simulink model "Copy_of_AB_Final_of_MPC_Bandwidth_Result"  (R2022b)
settings: Solver=FixedStepDiscrete  StartTime=0.0  StopTime=Inf  FixedStep=100e-6  RelTol=1e-3  EnableMultiTasking=on
undefined symbols (not defined in the file): C28x, CPU1, CPU2, CurrentBypassValue, DiscIntNeverNeededParam, Down, GPTRIP1SEL, TZ1, Up
libraries: c2802xlib x31, simulink x22, dspstat3 x17, dspsigops x9, c2837xDlib x6, c280xlib x5, PID_Lib x2, c2000lib x1, spsAlphaBetaZerotoabcLib x1, spsAlphaBetaZerotodq0Lib x1
(part 4 of 8)

== system Copy_of_AB_Final_of_MPC_Bandwidth_Result/Subsystem1/AlphaBetaDutiesCalculation/DutiesCalculation ==
  MPCC_f32AlphaVoltageReference : Inport
  MPCC_f32BetaVoltageReference : Inport  Port=2
  MPCC_f32DCLinkVoltage : Inport  Port=3
  Duty_Sector1 : Subsystem
  Duty_Sector2 : Subsystem
  Duty_Sector3 : Subsystem
  Duty_Sector4 : Subsystem
  Duty_Sector5 : Subsystem
  Duty_Sector6 : Subsystem
  Gain : Gain  Gain=2/3
  Gain{1,4,17,22} (4 alike) : Gain  Gain=1/3
  Gain10 : Gain  Gain=-2/3
  Gain{2,11..12,19} (4 alike) : Gain  Gain=0
  Gain13 : Gain  Gain=-1/sqrt(3)
  Gain14 : Gain  Gain=-2/3
  Gain{5,8,15..16} (4 alike) : Gain  Gain=-1/3
  Gain18 : Gain  Gain=-1/sqrt(3)
  Gain21 : Gain  Gain=-1/sqrt(3)
  Gain23 : Gain  Gain=2/3
  Gain{3,6..7,9} (4 alike) : Gain  Gain=1/sqrt(3)
  MPCC_f32Duty_Sector1 : Outport
  MPCC_f32Duty_Sector2 : Outport  Port=2
  MPCC_f32Duty_Sector3 : Outport  Port=3
  MPCC_f32Duty_Sector4 : Outport  Port=4
  MPCC_f32Duty_Sector5 : Outport  Port=5
  MPCC_f32Duty_Sector6 : Outport  Port=6
  wires:
  Duty_Sector1/1(MPCC_f32Duty_Sector1) -> MPCC_f32Duty_Sector1/1
  MPCC_f32DCLinkVoltage/1 -> [MPCC_f32DCLinkVoltage]
  Gain/1 -> Duty_Sector1/3(MPCC_f32AlphaConvVoltage1)
  [MPCC_f32DCLinkVoltage] -> Gain2/1, Gain3/1, Gain1/1, Gain/1
  Gain1/1 -> Duty_Sector1/4(MPCC_f32AlphaConvVoltage2)
  Gain2/1 -> Duty_Sector1/5(MPCC_f32BetaConvVoltage1)
  Gain3/1 -> Duty_Sector1/6(MPCC_f32BetaConvVoltage2)
  Duty_Sector2/1(MPCC_f32Duty_Sector2) -> MPCC_f32Duty_Sector2/1
  Gain7/1 -> Duty_Sector2/6(MPCC_f32BetaConvVoltage3)
  Gain4/1 -> Duty_Sector2/3(MPCC_f32AlphaConvVoltage2)
  Gain5/1 -> Duty_Sector2/4(MPCC_f32AlphaConvVoltage3)
  [MPCC_f32DCLinkVoltage] -> Gain6/1, Gain7/1, Gain5/1, Gain4/1
  [MPCC_f32DCLinkVoltage] -> Gain11/1, Gain9/1, Gain10/1, Gain8/1
  Duty_Sector3/1(MPCC_f32Duty_Sector3) -> MPCC_f32Duty_Sector3/1
  Duty_Sector4/1(MPCC_f32Duty_Sector4) -> MPCC_f32Duty_Sector4/1
  Gain13/1 -> Duty_Sector4/6(MPCC_f32BetaConvVoltage5)
  [MPCC_f32DCLinkVoltage] -> Gain12/1, Gain13/1, Gain15/1, Gain14/1
  Duty_Sector5/1(MPCC_f32Duty_Sector5) -> MPCC_f32Duty_Sector5/1
  [MPCC_f32DCLinkVoltage] -> Gain18/1, Gain17/1, Gain16/1
  Duty_Sector6/1(MPCC_f32Duty_Sector6) -> MPCC_f32Duty_Sector6/1
  Gain21/1 -> Duty_Sector6/5(MPCC_f32BetaConvVoltage6)
  [MPCC_f32DCLinkVoltage] -> Gain19/1, Gain21/1, Gain23/1, Gain22/1
  MPCC_f32AlphaVoltageReference/1 -> [MPCC_f32AlphaVoltageReference]
  MPCC_f32BetaVoltageReference/1 -> [MPCC_f32BetaVoltageReference]
  [MPCC_f32AlphaVoltageReference] -> Duty_Sector1/1(MPCC_f32AlphaVoltageReference)
  [MPCC_f32BetaVoltageReference] -> Duty_Sector1/2(MPCC_f32BetaVoltageReference)
  [MPCC_f32AlphaVoltageReference] -> Duty_Sector2/1(MPCC_f32AlphaVoltageReference)
  [MPCC_f32BetaVoltageReference] -> Duty_Sector2/2(MPCC_f32BetaVoltageReference)
  [MPCC_f32AlphaVoltageReference] -> Duty_Sector3/1(MPCC_f32AlphaVoltageReference)
  [MPCC_f32BetaVoltageReference] -> Duty_Sector3/2(MPCC_f32BetaVoltageReference)
  [MPCC_f32AlphaVoltageReference] -> Duty_Sector4/1(MPCC_f32AlphaVoltageReference)
  [MPCC_f32BetaVoltageReference] -> Duty_Sector4/2(MPCC_f32BetaVoltageReference)
  [MPCC_f32AlphaVoltageReference] -> Duty_Sector5/1(MPCC_f32AlphaVoltageReference)
  [MPCC_f32BetaVoltageReference] -> Duty_Sector5/2(MPCC_f32BetaVoltageReference)
  [MPCC_f32AlphaVoltageReference] -> Duty_Sector6/1(MPCC_f32AlphaVoltageReference)
  [MPCC_f32BetaVoltageReference] -> Duty_Sector6/2(MPCC_f32BetaVoltageReference)
  Gain6/1 -> Duty_Sector2/5(MPCC_f32BetaConvVoltage2)
  Gain8/1 -> Duty_Sector3/3(MPCC_f32AlphaConvVoltage3)
  Gain9/1 -> Duty_Sector3/5(MPCC_f32BetaConvVoltage3)
  Gain10/1 -> Duty_Sector3/4(MPCC_f32AlphaConvVoltage4)
  Gain11/1 -> Duty_Sector3/6(MPCC_f32BetaConvVoltage4)
  Gain14/1 -> Duty_Sector4/3(MPCC_f32AlphaConvVoltage4)
  Gain12/1 -> Duty_Sector4/5(MPCC_f32BetaConvVoltage4)
  Gain15/1 -> Duty_Sector4/4(MPCC_f32AlphaConvVoltage5)
  Gain18/1 -> Duty_Sector5/5(MPCC_f32BetaConvVoltage5), Duty_Sector5/6(MPCC_f32BetaConvVoltage6)
  Gain16/1 -> Duty_Sector5/3(MPCC_f32AlphaConvVoltage5)
  Gain17/1 -> Duty_Sector5/4(MPCC_f32AlphaConvVoltage6)
  Gain22/1 -> Duty_Sector6/3(MPCC_f32AlphaConvVoltage6)
  Gain23/1 -> Duty_Sector6/4(MPCC_f32AlphaConvVoltage1)
  Gain19/1 -> Duty_Sector6/6(MPCC_f32BetaConvVoltage1)

== system Copy_of_AB_Final_of_MPC_Bandwidth_Result/Subsystem1/GridCurrentFirstPrediction/PredictedIdGridCurrentCalculation ==
  MPCC_f32Predictionterm_A : Inport
  MPCC_f32Predictionterm_B : Inport  Port=2
  MPCC_f32Predictionterm_C : Inport  Port=3
  MPCC_f32DGridCurrent : Inport  Port=4
  MPCC_f32QGridCurrent : Inport  Port=5
  MPCC_f32DGridVoltage : Inport  Port=6
  MPCC_f32DConvVoltage : Inport  Port=7
  Add : Sum  Inputs=+++-
  Gain : Gain  Gain=0
  Product{,1..2,4} (4 alike) : Product
  MPCC_f32DGridCurrent_K_1 : Outport
  wires:
  Product/1 -> Add/1
  [MPCC_f32QGridCurrent] -> Product1/2
  [MPCC_f32Predictionterm_A] -> Product/1
  Product1/1 -> Gain/1
  [MPCC_f32DGridVoltage] -> Product2/2
  [MPCC_f32DGridCurrent] -> Product/2
  [MPCC_f32Predictionterm_C] -> Product1/1
  [MPCC_f32Predictionterm_B] -> Product2/1
  MPCC_f32Predictionterm_A/1 -> [MPCC_f32Predictionterm_A]
  MPCC_f32Predictionterm_B/1 -> [MPCC_f32Predictionterm_B]
  MPCC_f32Predictionterm_C/1 -> [MPCC_f32Predictionterm_C]
  MPCC_f32DGridCurrent/1 -> [MPCC_f32DGridCurrent]
  MPCC_f32QGridCurrent/1 -> [MPCC_f32QGridCurrent]
  MPCC_f32DGridVoltage/1 -> [MPCC_f32DGridVoltage]
  MPCC_f32DConvVoltage/1 -> [MPCC_f32DConvVoltage]
  Add/1 -> MPCC_f32DGridCurrent_K_1/1
  [MPCC_f32Predictionterm_B] -> Product4/1
  [MPCC_f32DConvVoltage] -> Product4/2
  Product2/1 -> Add/3
  Product4/1 -> Add/4
  Gain/1 -> Add/2

== system Copy_of_AB_Final_of_MPC_Bandwidth_Result/Subsystem1/GridCurrentFirstPrediction/PredictedIqGridCurrentCalculation ==
  MPCC_f32Predictionterm_A : Inport
  MPCC_f32Predictionterm_B : Inport  Port=2
  MPCC_f32Predictionterm_C : Inport  Port=3
  MPCC_f32DGridCurrent : Inport  Port=4
  MPCC_f32QGridCurrent : Inport  Port=5
  MPCC_f32QGridVoltage : Inport  Port=6
  MPCC_f32QConvVoltage : Inport  Port=7
  Add : Sum  Inputs=+-+-
  Gain : Gain  Gain=0
  Product : Product  OutDataTypeStr=Inherit: Inherit via back propagation
  Product1 : Product
  Product2 : Product
  Product4 : Product
  MPCC_f32QVoltageReference : Outport
  wires:
  Product/1 -> Add/1
  [MPCC_f32DGridCurrent] -> Product1/2
  [MPCC_f32Predictionterm_A] -> Product/1
  Product1/1 -> Gain/1
  [MPCC_f32QGridVoltage] -> Product2/2
  [MPCC_f32QGridCurrent] -> Product/2
  [MPCC_f32Predictionterm_C] -> Product1/1
  [MPCC_f32Predictionterm_B] -> Product2/1
  MPCC_f32Predictionterm_A/1 -> [MPCC_f32Predictionterm_A]
  MPCC_f32Predictionterm_B/1 -> [MPCC_f32Predictionterm_B]
  MPCC_f32Predictionterm_C/1 -> [MPCC_f32Predictionterm_C]
  MPCC_f32DGridCurrent/1 -> [MPCC_f32DGridCurrent]
  MPCC_f32QGridCurrent/1 -> [MPCC_f32QGridCurrent]
  MPCC_f32QGridVoltage/1 -> [MPCC_f32QGridVoltage]
  MPCC_f32QConvVoltage/1 -> [MPCC_f32QConvVoltage]
  Add/1 -> MPCC_f32QVoltageReference/1
  [MPCC_f32Predictionterm_B] -> Product4/1
  [MPCC_f32QConvVoltage] -> Product4/2
  Product2/1 -> Add/3
  Product4/1 -> Add/4
  Gain/1 -> Add/2

== system Copy_of_AB_Final_of_MPC_Bandwidth_Result/Subsystem1/GridCurrentSecondPrediction/CostFunctionofSectors ==
  MPCC_f32CostFunction_Voltage1 : Inport
  MPCC_f32CostFunction_Voltage2 : Inport  Port=2
  MPCC_f32CostFunction_Voltage3 : Inport  Port=3
  MPCC_f32CostFunction_Voltage4 : Inport  Port=4
  MPCC_f32CostFunction_Voltage5 : Inport  Port=5
  MPCC_f32CostFunction_Voltage6 : Inport  Port=6
  MPCC_f32Duty_Sector1 : Inport  Port=7
  MPCC_f32Duty_Sector2 : Inport  Port=8
  MPCC_f32Duty_Sector3 : Inport  Port=9
  MPCC_f32Duty_Sector4 : Inport  Port=10
  MPCC_f32Duty_Sector5 : Inport  Port=11
  MPCC_f32Duty_Sector6 : Inport  Port=12
  Duty_Sector1 : Subsystem
  Duty_Sector2 : Subsystem
  Duty_Sector3 : Subsystem
  Duty_Sector4 : Subsystem
  Duty_Sector5 : Subsystem
  Duty_Sector6 : Subsystem
  MPCC_f32CostFunction_Sector1 : Outport
  MPCC_f32CostFunction_Sector2 : Outport  Port=2
  MPCC_f32CostFunction_Sector3 : Outport  Port=3
  MPCC_f32CostFunction_Sector4 : Outport  Port=4
  MPCC_f32CostFunction_Sector5 : Outport  Port=5
  MPCC_f32CostFunction_Sector6 : Outport  Port=6
  wires:
  Duty_Sector1/1(MPCC_f32CostFunction_Sector1) -> MPCC_f32CostFunction_Sector1/1
  [MPCC_f32CostFunction_Voltage1] -> Duty_Sector1/1(MPCC_f32CostFunction_Voltage1)
  [MPCC_f32CostFunction_Voltage2] -> Duty_Sector1/2(MPCC_f32CostFunction_Voltage2)
  [MPCC_f32Duty_Sector1] -> Duty_Sector1/3(MPCC_f32Duty_Sector1)
  MPCC_f32Duty_Sector1/1 -> [MPCC_f32Duty_Sector1]
  MPCC_f32CostFunction_Voltage1/1 -> [MPCC_f32CostFunction_Voltage1]
  MPCC_f32CostFunction_Voltage2/1 -> [MPCC_f32CostFunction_Voltage2]
  MPCC_f32CostFunction_Voltage3/1 -> [MPCC_f32CostFunction_Voltage3]
  MPCC_f32CostFunction_Voltage4/1 -> [MPCC_f32CostFunction_Voltage4]
  MPCC_f32CostFunction_Voltage5/1 -> [MPCC_f32CostFunction_Voltage5]
  MPCC_f32CostFunction_Voltage6/1 -> [MPCC_f32CostFunction_Voltage6]
  MPCC_f32Duty_Sector2/1 -> [MPCC_f32Duty_Sector2]
  MPCC_f32Duty_Sector3/1 -> [MPCC_f32Duty_Sector3]
  MPCC_f32Duty_Sector4/1 -> [MPCC_f32Duty_Sector4]
  MPCC_f32Duty_Sector5/1 -> [MPCC_f32Duty_Sector5]
  MPCC_f32Duty_Sector6/1 -> [MPCC_f32Duty_Sector6]
  Duty_Sector2/1(MPCC_f32CostFunction_Sector2) -> MPCC_f32CostFunction_Sector2/1
  [MPCC_f32Duty_Sector2] -> Duty_Sector2/3(MPCC_f32Duty_Sector2)
  [MPCC_f32CostFunction_Voltage3] -> Duty_Sector2/2(MPCC_f32CostFunction_Voltage3)
  [MPCC_f32CostFunction_Voltage2] -> Duty_Sector2/1(MPCC_f32CostFunction_Voltage2)
  [MPCC_f32CostFunction_Voltage4] -> Duty_Sector3/2(MPCC_f32CostFunction_Voltage4)
  [MPCC_f32CostFunction_Voltage3] -> Duty_Sector3/1(MPCC_f32CostFunction_Voltage3)
  Duty_Sector3/1(MPCC_f32CostFunction_Sector3) -> MPCC_f32CostFunction_Sector3/1
  [MPCC_f32Duty_Sector3] -> Duty_Sector3/3(MPCC_f32Duty_Sector3)
  [MPCC_f32CostFunction_Voltage4] -> Duty_Sector4/1(MPCC_f32CostFunction_Voltage4)
  Duty_Sector4/1(MPCC_f32CostFunction_Sector4) -> MPCC_f32CostFunction_Sector4/1
  [MPCC_f32Duty_Sector4] -> Duty_Sector4/3(MPCC_f32Duty_Sector4)
  [MPCC_f32CostFunction_Voltage5] -> Duty_Sector4/2(MPCC_f32CostFunction_Voltage5)
  [MPCC_f32CostFunction_Voltage5] -> Duty_Sector5/1(MPCC_f32CostFunction_Voltage5)
  [MPCC_f32Duty_Sector5] -> Duty_Sector5/3(MPCC_f32Duty_Sector5)
  Duty_Sector5/1(MPCC_f32CostFunction_Sector5) -> MPCC_f32CostFunction_Sector5/1
  [MPCC_f32CostFunction_Voltage6] -> Duty_Sector5/2(MPCC_f32CostFunction_Voltage6)
  [MPCC_f32CostFunction_Voltage1] -> Duty_Sector6/2(MPCC_f32CostFunction_Voltage1)
  [MPCC_f32Duty_Sector6] -> Duty_Sector6/3(MPCC_f32Duty_Sector6)
  Duty_Sector6/1(MPCC_f32CostFunction_Sector6) -> MPCC_f32CostFunction_Sector6/1
  [MPCC_f32CostFunction_Voltage6] -> Duty_Sector6/1(MPCC_f32CostFunction_Voltage6)

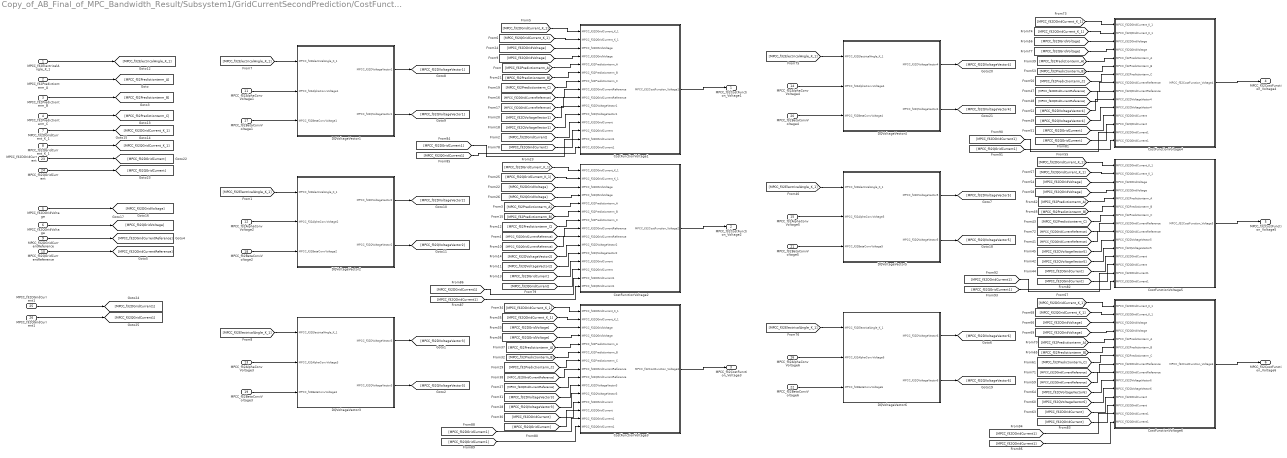
== system Copy_of_AB_Final_of_MPC_Bandwidth_Result/Subsystem1/GridCurrentSecondPrediction/CostFunctionofVoltageVectors ==
  MPCC_f32ElectricalAngle_K_1 : Inport
  MPCC_f32Predictionterm_A : Inport  Port=2
  MPCC_f32Predictionterm_B : Inport  Port=3
  MPCC_f32Predictionterm_C : Inport  Port=4
  MPCC_f32DGridVoltage : Inport  Port=5
  MPCC_f32QGridVoltage : Inport  Port=6
  MPCC_f32DGridCurrent_K_1 : Inport  Port=7
  MPCC_f32QGridCurrent_K_1 : Inport  Port=8
  MPCC_f32DGridCurrentReference : Inport  Port=9
  MPCC_f32QGridCurrentReference : Inport  Port=10
  MPCC_f32AlphaConvVoltage1 : Inport  Port=11
  MPCC_f32AlphaConvVoltage2 : Inport  Port=12
  MPCC_f32AlphaConvVoltage3 : Inport  Port=13
  MPCC_f32AlphaConvVoltage4 : Inport  Port=14
  MPCC_f32AlphaConvVoltage5 : Inport  Port=15
  MPCC_f32AlphaConvVoltage6 : Inport  Port=16
  MPCC_f32BetaConvVoltage1 : Inport  Port=17
  MPCC_f32BetaConvVoltage2 : Inport  Port=18
  MPCC_f32BetaConvVoltage3 : Inport  Port=19
  MPCC_f32BetaConvVoltage4 : Inport  Port=20
  MPCC_f32BetaConvVoltage5 : Inport  Port=21
  MPCC_f32BetaConvVoltage6 : Inport  Port=22
  MPCC_f32DGridCurrent : Inport  Port=23
  MPCC_f32QGridCurrent : Inport  Port=24
  MPCC_f32DGridCurrent1 : Inport  Port=25
  MPCC_f32QGridCurrent1 : Inport  Port=26
  CostFunctionVoltage1 : Subsystem
  CostFunctionVoltage2 : Subsystem
  CostFunctionVoltage3 : Subsystem
  CostFunctionVoltage4 : Subsystem
  CostFunctionVoltage5 : Subsystem
  CostFunctionVoltage6 : Subsystem
  DQVoltageVector1 : Subsystem
  DQVoltageVector2 : Subsystem
  DQVoltageVector3 : Subsystem
  DQVoltageVector4 : Subsystem
  DQVoltageVector5 : Subsystem
  DQVoltageVector6 : Subsystem
  MPCC_f32CostFunction_Voltage1 : Outport
  MPCC_f32CostFunction_Voltage2 : Outport  Port=2
  MPCC_f32CostFunction_Voltage3 : Outport  Port=3
  MPCC_f32CostFunction_Voltage4 : Outport  Port=4
  MPCC_f32CostFunction_Voltage5 : Outport  Port=5
  MPCC_f32CostFunction_Voltage6 : Outport  Port=6
  wires:
  DQVoltageVector1/1(MPCC_f32DVoltageVector1) -> [MPCC_f32DVoltageVector1]
  DQVoltageVector1/2(MPCC_f32QVoltageVector1) -> [MPCC_f32QVoltageVector1]
  DQVoltageVector2/1(MPCC_f32DVoltageVector2) -> [MPCC_f32DVoltageVector2]
  DQVoltageVector2/2(MPCC_f32QVoltageVector2) -> [MPCC_f32QVoltageVector2]
  [MPCC_f32ElectricalAngle_K_1] -> DQVoltageVector1/1(MPCC_f32ElectricalAngle_K_1)
  [MPCC_f32ElectricalAngle_K_1] -> DQVoltageVector2/1(MPCC_f32ElectricalAngle_K_1)
  MPCC_f32AlphaConvVoltage1/1 -> DQVoltageVector1/2(MPCC_f32AlphaConvVoltage1)
  MPCC_f32BetaConvVoltage1/1 -> DQVoltageVector1/3(MPCC_f32BetaConvVoltage1)
  MPCC_f32AlphaConvVoltage2/1 -> DQVoltageVector2/2(MPCC_f32AlphaConvVoltage2)
  MPCC_f32BetaConvVoltage2/1 -> DQVoltageVector2/3(MPCC_f32BetaConvVoltage2)
  MPCC_f32ElectricalAngle_K_1/1 -> [MPCC_f32ElectricalAngle_K_1]
  MPCC_f32DGridVoltage/1 -> [MPCC_f32DGridVoltage]
  MPCC_f32QGridCurrent_K_1/1 -> [MPCC_f32QGridCurrent_K_1]
  MPCC_f32DGridCurrent_K_1/1 -> [MPCC_f32DGridCurrent_K_1]
  MPCC_f32QGridVoltage/1 -> [MPCC_f32QGridVoltage]
  MPCC_f32Predictionterm_B/1 -> [MPCC_f32Predictionterm_B]
  MPCC_f32Predictionterm_C/1 -> [MPCC_f32Predictionterm_C]
  MPCC_f32Predictionterm_A/1 -> [MPCC_f32Predictionterm_A]
  MPCC_f32DGridCurrentReference/1 -> [MPCC_f32DGridCurrentReference]
  MPCC_f32QGridCurrentReference/1 -> [MPCC_f32QGridCurrentReference]
  CostFunctionVoltage1/1(MPCC_f32CostFunction_Voltage1) -> MPCC_f32CostFunction_Voltage1/1
  CostFunctionVoltage2/1(MPCC_f32CostFunction_Voltage2) -> MPCC_f32CostFunction_Voltage2/1
  [MPCC_f32DGridCurrent_K_1] -> CostFunctionVoltage1/1(MPCC_f32DGridCurrent_K_1)
  [MPCC_f32QGridCurrent_K_1] -> CostFunctionVoltage1/2(MPCC_f32QGridCurrent_K_1)
  [MPCC_f32DGridVoltage] -> CostFunctionVoltage1/3(MPCC_f32DGridVoltage)
  [MPCC_f32QGridVoltage] -> CostFunctionVoltage1/4(MPCC_f32QGridVoltage)
  [MPCC_f32Predictionterm_A] -> CostFunctionVoltage1/5(MPCC_f32Predictionterm_A)
  [MPCC_f32Predictionterm_B] -> CostFunctionVoltage1/6(MPCC_f32Predictionterm_B)
  [MPCC_f32Predictionterm_C] -> CostFunctionVoltage1/7(MPCC_f32Predictionterm_C)
  [MPCC_f32DGridCurrentReference] -> CostFunctionVoltage1/8(MPCC_f32DGridCurrentReference)
  [MPCC_f32QGridCurrentReference] -> CostFunctionVoltage1/9(MPCC_f32QGridCurrentReference)
  [MPCC_f32DVoltageVector1] -> CostFunctionVoltage1/10(MPCC_f32DVoltageVector1)
  [MPCC_f32QVoltageVector1] -> CostFunctionVoltage1/11(MPCC_f32QVoltageVector1)
  [MPCC_f32Predictionterm_C] -> CostFunctionVoltage2/7(MPCC_f32Predictionterm_C)
  [MPCC_f32DGridCurrentReference] -> CostFunctionVoltage2/8(MPCC_f32DGridCurrentReference)
  [MPCC_f32QGridCurrentReference] -> CostFunctionVoltage2/9(MPCC_f32QGridCurrentReference)
  [MPCC_f32DVoltageVector2] -> CostFunctionVoltage2/10(MPCC_f32DVoltageVector2)
  [MPCC_f32QVoltageVector2] -> CostFunctionVoltage2/11(MPCC_f32QVoltageVector2)
  [MPCC_f32QGridCurrent_K_1] -> CostFunctionVoltage2/2(MPCC_f32QGridCurrent_K_1)
  [MPCC_f32DGridVoltage] -> CostFunctionVoltage2/3(MPCC_f32DGridVoltage)
  [MPCC_f32QGridVoltage] -> CostFunctionVoltage2/4(MPCC_f32QGridVoltage)
  [MPCC_f32Predictionterm_A] -> CostFunctionVoltage2/5(MPCC_f32Predictionterm_A)
  [MPCC_f32Predictionterm_B] -> CostFunctionVoltage2/6(MPCC_f32Predictionterm_B)
  [MPCC_f32DGridCurrent_K_1] -> CostFunctionVoltage2/1(MPCC_f32DGridCurrent_K_1)
  MPCC_f32BetaConvVoltage3/1 -> DQVoltageVector3/3(MPCC_f32BetaConvVoltage3)
  MPCC_f32AlphaConvVoltage3/1 -> DQVoltageVector3/2(MPCC_f32AlphaConvVoltage3)
  [MPCC_f32ElectricalAngle_K_1] -> DQVoltageVector3/1(MPCC_f32ElectricalAngle_K_1)
  DQVoltageVector3/1(MPCC_f32DVoltageVector3) -> [MPCC_f32DVoltageVector3]
  DQVoltageVector3/2(MPCC_f32QVoltageVector3) -> [MPCC_f32QVoltageVector3]
  CostFunctionVoltage3/1(MPCC_f32CostFunction_Voltage3) -> MPCC_f32CostFunction_Voltage3/1
  [MPCC_f32Predictionterm_A] -> CostFunctionVoltage3/5(MPCC_f32Predictionterm_A)
  [MPCC_f32QGridVoltage] -> CostFunctionVoltage3/4(MPCC_f32QGridVoltage)
  [MPCC_f32Predictionterm_B] -> CostFunctionVoltage3/6(MPCC_f32Predictionterm_B)
  [MPCC_f32QGridCurrent_K_1] -> CostFunctionVoltage3/2(MPCC_f32QGridCurrent_K_1)
  [MPCC_f32QVoltageVector3] -> CostFunctionVoltage3/11(MPCC_f32QVoltageVector3)
  [MPCC_f32DVoltageVector3] -> CostFunctionVoltage3/10(MPCC_f32DVoltageVector3)
  [MPCC_f32DGridVoltage] -> CostFunctionVoltage3/3(MPCC_f32DGridVoltage)
  [MPCC_f32Predictionterm_C] -> CostFunctionVoltage3/7(MPCC_f32Predictionterm_C)
  [MPCC_f32QGridCurrentReference] -> CostFunctionVoltage3/9(MPCC_f32QGridCurrentReference)
  [MPCC_f32DGridCurrent_K_1] -> CostFunctionVoltage3/1(MPCC_f32DGridCurrent_K_1)
  [MPCC_f32DGridCurrentReference] -> CostFunctionVoltage3/8(MPCC_f32DGridCurrentReference)
  [MPCC_f32DGridVoltage] -> CostFunctionVoltage4/3(MPCC_f32DGridVoltage)
  [MPCC_f32Predictionterm_C] -> CostFunctionVoltage4/7(MPCC_f32Predictionterm_C)
  [MPCC_f32Predictionterm_B] -> CostFunctionVoltage4/6(MPCC_f32Predictionterm_B)
  [MPCC_f32QGridCurrent_K_1] -> CostFunctionVoltage4/2(MPCC_f32QGridCurrent_K_1)
  [MPCC_f32DGridCurrent_K_1] -> CostFunctionVoltage4/1(MPCC_f32DGridCurrent_K_1)
  [MPCC_f32Predictionterm_A] -> CostFunctionVoltage4/5(MPCC_f32Predictionterm_A)
  [MPCC_f32QGridVoltage] -> CostFunctionVoltage5/4(MPCC_f32QGridVoltage)
  [MPCC_f32Predictionterm_B] -> CostFunctionVoltage5/6(MPCC_f32Predictionterm_B)
  [MPCC_f32QGridCurrent_K_1] -> CostFunctionVoltage5/2(MPCC_f32QGridCurrent_K_1)
  [MPCC_f32DVoltageVector5] -> CostFunctionVoltage5/10(MPCC_f32DVoltageVector5)
  [MPCC_f32Predictionterm_C] -> CostFunctionVoltage5/7(MPCC_f32Predictionterm_C)
  [MPCC_f32DGridCurrentReference] -> CostFunctionVoltage5/8(MPCC_f32DGridCurrentReference)
  [MPCC_f32QGridCurrentReference] -> CostFunctionVoltage5/9(MPCC_f32QGridCurrentReference)
  [MPCC_f32DGridCurrent_K_1] -> CostFunctionVoltage5/1(MPCC_f32DGridCurrent_K_1)
  [MPCC_f32DVoltageVector4] -> CostFunctionVoltage4/10(MPCC_f32DVoltageVector4)
  [MPCC_f32QGridCurrentReference] -> CostFunctionVoltage6/9(MPCC_f32QGridCurrentReference)
  [MPCC_f32QVoltageVector5] -> CostFunctionVoltage5/11(MPCC_f32QVoltageVector5)
  [MPCC_f32DGridCurrentReference] -> CostFunctionVoltage6/8(MPCC_f32DGridCurrentReference)
  CostFunctionVoltage4/1(MPCC_f32CostFunction_Voltage4) -> MPCC_f32CostFunction_Voltage4/1
  [MPCC_f32DVoltageVector6] -> CostFunctionVoltage6/10(MPCC_f32DVoltageVector6)
  [MPCC_f32DGridVoltage] -> CostFunctionVoltage6/3(MPCC_f32DGridVoltage)
  [MPCC_f32Predictionterm_C] -> CostFunctionVoltage6/7(MPCC_f32Predictionterm_C)
  [MPCC_f32QGridVoltage] -> CostFunctionVoltage4/4(MPCC_f32QGridVoltage)
  [MPCC_f32QGridCurrent_K_1] -> CostFunctionVoltage6/2(MPCC_f32QGridCurrent_K_1)
  [MPCC_f32QVoltageVector6] -> CostFunctionVoltage6/11(MPCC_f32QVoltageVector6)
  [MPCC_f32Predictionterm_B] -> CostFunctionVoltage6/6(MPCC_f32Predictionterm_B)
  CostFunctionVoltage5/1(MPCC_f32CostFunction_Voltage5) -> MPCC_f32CostFunction_Voltage5/1
  [MPCC_f32QGridVoltage] -> CostFunctionVoltage6/4(MPCC_f32QGridVoltage)
  MPCC_f32AlphaConvVoltage6/1 -> DQVoltageVector6/2(MPCC_f32AlphaConvVoltage6)
  [MPCC_f32Predictionterm_A] -> CostFunctionVoltage5/5(MPCC_f32Predictionterm_A)
  DQVoltageVector6/1(MPCC_f32DVoltageVector6) -> [MPCC_f32DVoltageVector6]
  [MPCC_f32DGridVoltage] -> CostFunctionVoltage5/3(MPCC_f32DGridVoltage)
  MPCC_f32BetaConvVoltage6/1 -> DQVoltageVector6/3(MPCC_f32BetaConvVoltage6)
  DQVoltageVector6/2(MPCC_f32QVoltageVector6) -> [MPCC_f32QVoltageVector6]
  [MPCC_f32ElectricalAngle_K_1] -> DQVoltageVector4/1(MPCC_f32ElectricalAngle_K_1)
  DQVoltageVector5/2(MPCC_f32QVoltageVector5) -> [MPCC_f32QVoltageVector5]
  CostFunctionVoltage6/1(MPCC_f32CostFunction_Voltage6) -> MPCC_f32CostFunction_Voltage6/1
  MPCC_f32AlphaConvVoltage5/1 -> DQVoltageVector5/2(MPCC_f32AlphaConvVoltage5)
  DQVoltageVector4/1(MPCC_f32DVoltageVector4) -> [MPCC_f32DVoltageVector4]
  [MPCC_f32Predictionterm_A] -> CostFunctionVoltage6/5(MPCC_f32Predictionterm_A)
  DQVoltageVector4/2(MPCC_f32QVoltageVector4) -> [MPCC_f32QVoltageVector4]
  [MPCC_f32ElectricalAngle_K_1] -> DQVoltageVector5/1(MPCC_f32ElectricalAngle_K_1)
  MPCC_f32BetaConvVoltage4/1 -> DQVoltageVector4/3(MPCC_f32BetaConvVoltage4)
  [MPCC_f32QVoltageVector4] -> CostFunctionVoltage4/11(MPCC_f32QVoltageVector4)
  DQVoltageVector5/1(MPCC_f32DVoltageVector5) -> [MPCC_f32DVoltageVector5]
  [MPCC_f32QGridCurrentReference] -> CostFunctionVoltage4/9(MPCC_f32QGridCurrentReference)
  [MPCC_f32ElectricalAngle_K_1] -> DQVoltageVector6/1(MPCC_f32ElectricalAngle_K_1)
  [MPCC_f32DGridCurrent_K_1] -> CostFunctionVoltage6/1(MPCC_f32DGridCurrent_K_1)
  MPCC_f32AlphaConvVoltage4/1 -> DQVoltageVector4/2(MPCC_f32AlphaConvVoltage4)
  MPCC_f32BetaConvVoltage5/1 -> DQVoltageVector5/3(MPCC_f32BetaConvVoltage5)
  [MPCC_f32DGridCurrentReference] -> CostFunctionVoltage4/8(MPCC_f32DGridCurrentReference)
  [MPCC_f32DGridCurrent] -> CostFunctionVoltage1/12(MPCC_f32DGridCurrent)
  [MPCC_f32QGridCurrent] -> CostFunctionVoltage1/13(MPCC_f32QGridCurrent)
  MPCC_f32DGridCurrent/1 -> [MPCC_f32DGridCurrent]
  MPCC_f32QGridCurrent/1 -> [MPCC_f32QGridCurrent]
  [MPCC_f32DGridCurrent] -> CostFunctionVoltage2/12(MPCC_f32DGridCurrent)
  [MPCC_f32QGridCurrent] -> CostFunctionVoltage2/13(MPCC_f32QGridCurrent)
  [MPCC_f32DGridCurrent] -> CostFunctionVoltage3/12(MPCC_f32DGridCurrent)
  [MPCC_f32QGridCurrent] -> CostFunctionVoltage3/13(MPCC_f32QGridCurrent)
  [MPCC_f32DGridCurrent] -> CostFunctionVoltage4/12(MPCC_f32DGridCurrent)
  [MPCC_f32QGridCurrent] -> CostFunctionVoltage4/13(MPCC_f32QGridCurrent)
  [MPCC_f32DGridCurrent] -> CostFunctionVoltage5/12(MPCC_f32DGridCurrent)
  [MPCC_f32QGridCurrent] -> CostFunctionVoltage5/13(MPCC_f32QGridCurrent)
  [MPCC_f32DGridCurrent] -> CostFunctionVoltage6/12(MPCC_f32DGridCurrent)
  [MPCC_f32QGridCurrent] -> CostFunctionVoltage6/13(MPCC_f32QGridCurrent)
  MPCC_f32QGridCurrent1/1 -> [MPCC_f32QGridCurrent1]
  MPCC_f32DGridCurrent1/1 -> [MPCC_f32DGridCurrent1]
  [MPCC_f32DGridCurrent1] -> CostFunctionVoltage1/14(MPCC_f32DGridCurrent1)
  [MPCC_f32QGridCurrent1] -> CostFunctionVoltage1/15(MPCC_f32QGridCurrent1)
  [MPCC_f32DGridCurrent1] -> CostFunctionVoltage2/14(MPCC_f32DGridCurrent1)
  [MPCC_f32QGridCurrent1] -> CostFunctionVoltage2/15(MPCC_f32QGridCurrent1)
  [MPCC_f32DGridCurrent1] -> CostFunctionVoltage3/14(MPCC_f32DGridCurrent1)
  [MPCC_f32QGridCurrent1] -> CostFunctionVoltage3/15(MPCC_f32QGridCurrent1)
  [MPCC_f32DGridCurrent1] -> CostFunctionVoltage4/14(MPCC_f32DGridCurrent1)
  [MPCC_f32QGridCurrent1] -> CostFunctionVoltage4/15(MPCC_f32QGridCurrent1)
  [MPCC_f32DGridCurrent1] -> CostFunctionVoltage5/14(MPCC_f32DGridCurrent1)
  [MPCC_f32QGridCurrent1] -> CostFunctionVoltage5/15(MPCC_f32QGridCurrent1)
  [MPCC_f32DGridCurrent1] -> CostFunctionVoltage6/14(MPCC_f32DGridCurrent1)
  [MPCC_f32QGridCurrent1] -> CostFunctionVoltage6/15(MPCC_f32QGridCurrent1)

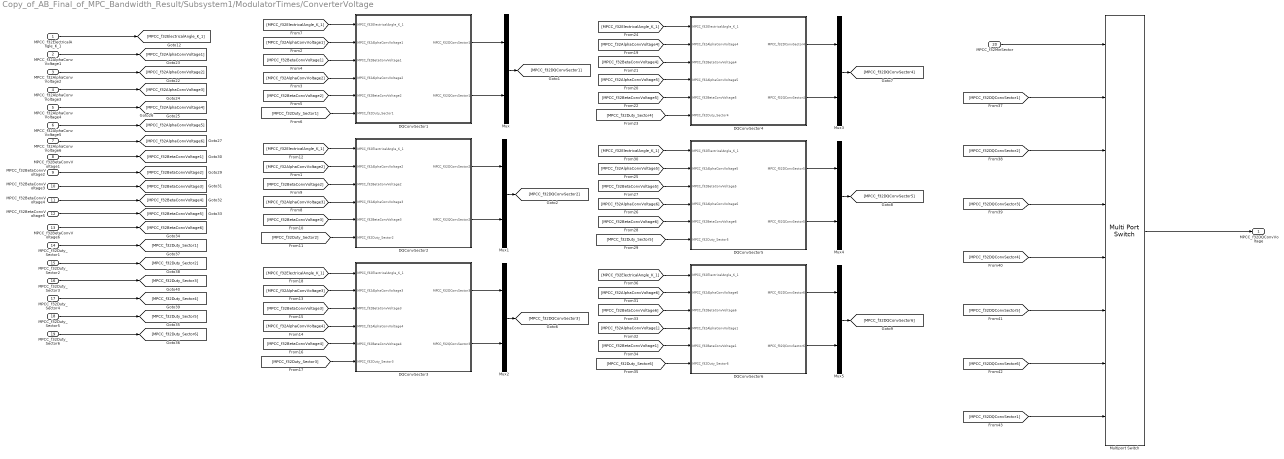
== system Copy_of_AB_Final_of_MPC_Bandwidth_Result/Subsystem1/ModulatorTimes/ConverterVoltage ==
  MPCC_f32ElectricalAngle_K_1 : Inport
  MPCC_f32AlphaConvVoltage1 : Inport  Port=2
  MPCC_f32AlphaConvVoltage2 : Inport  Port=3
  MPCC_f32AlphaConvVoltage3 : Inport  Port=4
  MPCC_f32AlphaConvVoltage4 : Inport  Port=5
  MPCC_f32AlphaConvVoltage5 : Inport  Port=6
  MPCC_f32AlphaConvVoltage6 : Inport  Port=7
  MPCC_f32BetaConvVoltage1 : Inport  Port=8
  MPCC_f32BetaConvVoltage2 : Inport  Port=9
  MPCC_f32BetaConvVoltage3 : Inport  Port=10
  MPCC_f32BetaConvVoltage4 : Inport  Port=11
  MPCC_f32BetaConvVoltage5 : Inport  Port=12
  MPCC_f32BetaConvVoltage6 : Inport  Port=13
  MPCC_f32Duty_Sector1 : Inport  Port=14
  MPCC_f32Duty_Sector2 : Inport  Port=15
  MPCC_f32Duty_Sector3 : Inport  Port=16
  MPCC_f32Duty_Sector4 : Inport  Port=17
  MPCC_f32Duty_Sector5 : Inport  Port=18
  MPCC_f32Duty_Sector6 : Inport  Port=19
  MPCC_f32MinSector : Inport  Port=20
  DQConvSector1 : Subsystem
  DQConvSector2 : Subsystem
  DQConvSector3 : Subsystem
  DQConvSector4 : Subsystem
  DQConvSector5 : Subsystem
  DQConvSector6 : Subsystem
  Multiport Switch : MultiPortSwitch  Inputs=6  DataPortForDefault=Additional data port  DiagnosticForDefault=None  SaturateOnIntegerOverflow=off  InputSameDT=off
  Mux{,1..5} (6 alike) : Mux  Inputs=2
  MPCC_f32DQConvVoltage : Outport
  wires:
  DQConvSector1/1(MPCC_f32DConvSector1) -> Mux/1
  DQConvSector1/2(MPCC_f32QConvSector1) -> Mux/2
  [MPCC_f32ElectricalAngle_K_1] -> DQConvSector1/1(MPCC_f32ElectricalAngle_K_1)
  MPCC_f32ElectricalAngle_K_1/1 -> [MPCC_f32ElectricalAngle_K_1]
  MPCC_f32AlphaConvVoltage1/1 -> [MPCC_f32AlphaConvVoltage1]
  MPCC_f32AlphaConvVoltage2/1 -> [MPCC_f32AlphaConvVoltage2]
  MPCC_f32AlphaConvVoltage3/1 -> [MPCC_f32AlphaConvVoltage3]
  MPCC_f32AlphaConvVoltage4/1 -> [MPCC_f32AlphaConvVoltage4]
  MPCC_f32AlphaConvVoltage5/1 -> [MPCC_f32AlphaConvVoltage5]
  MPCC_f32AlphaConvVoltage6/1 -> [MPCC_f32AlphaConvVoltage6]
  MPCC_f32BetaConvVoltage1/1 -> [MPCC_f32BetaConvVoltage1]
  MPCC_f32BetaConvVoltage2/1 -> [MPCC_f32BetaConvVoltage2]
  MPCC_f32BetaConvVoltage3/1 -> [MPCC_f32BetaConvVoltage3]
  MPCC_f32BetaConvVoltage4/1 -> [MPCC_f32BetaConvVoltage4]
  MPCC_f32BetaConvVoltage5/1 -> [MPCC_f32BetaConvVoltage5]
  MPCC_f32BetaConvVoltage6/1 -> [MPCC_f32BetaConvVoltage6]
  MPCC_f32Duty_Sector2/1 -> [MPCC_f32Duty_Sector2]
  MPCC_f32Duty_Sector4/1 -> [MPCC_f32Duty_Sector4]
  MPCC_f32Duty_Sector6/1 -> [MPCC_f32Duty_Sector6]
  MPCC_f32Duty_Sector1/1 -> [MPCC_f32Duty_Sector1]
  MPCC_f32Duty_Sector3/1 -> [MPCC_f32Duty_Sector3]
  MPCC_f32Duty_Sector5/1 -> [MPCC_f32Duty_Sector5]
  [MPCC_f32Duty_Sector1] -> DQConvSector1/6(MPCC_f32Duty_Sector1)
  [MPCC_f32AlphaConvVoltage1] -> DQConvSector1/2(MPCC_f32AlphaConvVoltage1)
  [MPCC_f32BetaConvVoltage1] -> DQConvSector1/3(MPCC_f32BetaConvVoltage1)
  [MPCC_f32AlphaConvVoltage2] -> DQConvSector1/4(MPCC_f32AlphaConvVoltage2)
  [MPCC_f32BetaConvVoltage2] -> DQConvSector1/5(MPCC_f32BetaConvVoltage2)
  [MPCC_f32AlphaConvVoltage3] -> DQConvSector2/4(MPCC_f32AlphaConvVoltage3)
  [MPCC_f32BetaConvVoltage3] -> DQConvSector2/5(MPCC_f32BetaConvVoltage3)
  [MPCC_f32BetaConvVoltage2] -> DQConvSector2/3(MPCC_f32BetaConvVoltage2)
  [MPCC_f32AlphaConvVoltage2] -> DQConvSector2/2(MPCC_f32AlphaConvVoltage2)
  [MPCC_f32Duty_Sector2] -> DQConvSector2/6(MPCC_f32Duty_Sector2)
  [MPCC_f32ElectricalAngle_K_1] -> DQConvSector2/1(MPCC_f32ElectricalAngle_K_1)
  [MPCC_f32AlphaConvVoltage4] -> DQConvSector3/4(MPCC_f32AlphaConvVoltage4)
  [MPCC_f32BetaConvVoltage4] -> DQConvSector3/5(MPCC_f32BetaConvVoltage4)
  [MPCC_f32BetaConvVoltage3] -> DQConvSector3/3(MPCC_f32BetaConvVoltage3)
  [MPCC_f32AlphaConvVoltage3] -> DQConvSector3/2(MPCC_f32AlphaConvVoltage3)
  [MPCC_f32Duty_Sector3] -> DQConvSector3/6(MPCC_f32Duty_Sector3)
  [MPCC_f32ElectricalAngle_K_1] -> DQConvSector3/1(MPCC_f32ElectricalAngle_K_1)
  [MPCC_f32AlphaConvVoltage5] -> DQConvSector4/4(MPCC_f32AlphaConvVoltage5)
  [MPCC_f32BetaConvVoltage5] -> DQConvSector4/5(MPCC_f32BetaConvVoltage5)
  [MPCC_f32BetaConvVoltage4] -> DQConvSector4/3(MPCC_f32BetaConvVoltage4)
  [MPCC_f32AlphaConvVoltage4] -> DQConvSector4/2(MPCC_f32AlphaConvVoltage4)
  [MPCC_f32Duty_Sector4] -> DQConvSector4/6(MPCC_f32Duty_Sector4)
  [MPCC_f32ElectricalAngle_K_1] -> DQConvSector4/1(MPCC_f32ElectricalAngle_K_1)
  [MPCC_f32AlphaConvVoltage6] -> DQConvSector5/4(MPCC_f32AlphaConvVoltage6)
  [MPCC_f32BetaConvVoltage6] -> DQConvSector5/5(MPCC_f32BetaConvVoltage6)
  [MPCC_f32BetaConvVoltage5] -> DQConvSector5/3(MPCC_f32BetaConvVoltage5)
  [MPCC_f32AlphaConvVoltage5] -> DQConvSector5/2(MPCC_f32AlphaConvVoltage5)
  [MPCC_f32Duty_Sector5] -> DQConvSector5/6(MPCC_f32Duty_Sector5)
  [MPCC_f32ElectricalAngle_K_1] -> DQConvSector5/1(MPCC_f32ElectricalAngle_K_1)
  [MPCC_f32AlphaConvVoltage1] -> DQConvSector6/4(MPCC_f32AlphaConvVoltage1)
  [MPCC_f32BetaConvVoltage1] -> DQConvSector6/5(MPCC_f32BetaConvVoltage1)
  [MPCC_f32BetaConvVoltage6] -> DQConvSector6/3(MPCC_f32BetaConvVoltage6)
  [MPCC_f32AlphaConvVoltage6] -> DQConvSector6/2(MPCC_f32AlphaConvVoltage6)
  [MPCC_f32Duty_Sector6] -> DQConvSector6/6(MPCC_f32Duty_Sector6)
  [MPCC_f32ElectricalAngle_K_1] -> DQConvSector6/1(MPCC_f32ElectricalAngle_K_1)
  Mux/1 -> [MPCC_f32DQConvSector1]
  Mux1/1 -> [MPCC_f32DQConvSector2]
  DQConvSector2/2(MPCC_f32QConvSector2) -> Mux1/2
  DQConvSector2/1(MPCC_f32DConvSector2) -> Mux1/1
  DQConvSector3/2(MPCC_f32QConvSector3) -> Mux2/2
  DQConvSector3/1(MPCC_f32DConvSector3) -> Mux2/1
  Mux2/1 -> [MPCC_f32DQConvSector3]
  DQConvSector4/2(MPCC_f32QConvSector4) -> Mux3/2
  DQConvSector4/1(MPCC_f32DConvSector4) -> Mux3/1
  Mux3/1 -> [MPCC_f32DQConvSector4]
  DQConvSector5/2(MPCC_f32QConvSector5) -> Mux4/2
  DQConvSector5/1(MPCC_f32DConvSector5) -> Mux4/1
  Mux4/1 -> [MPCC_f32DQConvSector5]
  DQConvSector6/2(MPCC_f32QConvSector6) -> Mux5/2
  DQConvSector6/1(MPCC_f32DConvSector6) -> Mux5/1
  Mux5/1 -> [MPCC_f32DQConvSector6]
  [MPCC_f32DQConvSector1] -> Multiport Switch/2
  [MPCC_f32DQConvSector2] -> Multiport Switch/3
  [MPCC_f32DQConvSector3] -> Multiport Switch/4
  [MPCC_f32DQConvSector4] -> Multiport Switch/5
  [MPCC_f32DQConvSector5] -> Multiport Switch/6
  [MPCC_f32DQConvSector6] -> Multiport Switch/7
  MPCC_f32MinSector/1 -> Multiport Switch/1
  [MPCC_f32DQConvSector1] -> Multiport Switch/8
  Multiport Switch/1 -> MPCC_f32DQConvVoltage/1

== system Copy_of_AB_Final_of_MPC_Bandwidth_Result/Subsystem1/ModulatorTimes/ModulationVectorTimes ==
  MPCC_f32Duty_Sector1 : Inport
  MPCC_f32Duty_Sector2 : Inport  Port=2
  MPCC_f32Duty_Sector3 : Inport  Port=3
  MPCC_f32Duty_Sector4 : Inport  Port=4
  MPCC_f32Duty_Sector5 : Inport  Port=5
  MPCC_f32Duty_Sector6 : Inport  Port=6
  MPCC_f32SwitchingPeriod : Inport  Port=7
  MPCC_f32MinSector : Inport  Port=8
  Demux : Demux
  Multiport Switch : MultiPortSwitch  Inputs=6  DataPortForDefault=Additional data port  DiagnosticForDefault=None  SaturateOnIntegerOverflow=off  InputSameDT=off
  Product : Product
  Product1 : Product
  Product2 : Product
  MPCC_f32Time1 : Outport
  MPCC_f32Time2 : Outport  Port=2
  MPCC_f32Time0 : Outport  Port=3
  MPCC_u8ModulationSector : Outport  Port=4
  wires:
  MPCC_f32Duty_Sector1/1 -> [MPCC_f32Duty_Sector1]
  MPCC_f32Duty_Sector2/1 -> [MPCC_f32Duty_Sector2]
  MPCC_f32Duty_Sector3/1 -> [MPCC_f32Duty_Sector3]
  MPCC_f32Duty_Sector4/1 -> [MPCC_f32Duty_Sector4]
  MPCC_f32Duty_Sector5/1 -> [MPCC_f32Duty_Sector5]
  MPCC_f32Duty_Sector6/1 -> [MPCC_f32Duty_Sector6]
  MPCC_f32SwitchingPeriod/1 -> [MPCC_f32SwitchingPeriod]
  MPCC_f32MinSector/1 -> [MPCC_f32MinSector]
  [MPCC_f32MinSector] -> Multiport Switch/1
  [MPCC_f32Duty_Sector1] -> Multiport Switch/2
  [MPCC_f32Duty_Sector2] -> Multiport Switch/3
  [MPCC_f32Duty_Sector3] -> Multiport Switch/4
  [MPCC_f32Duty_Sector4] -> Multiport Switch/5
  [MPCC_f32Duty_Sector5] -> Multiport Switch/6
  [MPCC_f32Duty_Sector6] -> Multiport Switch/7
  [MPCC_f32Duty_Sector1] -> Multiport Switch/8
  Multiport Switch/1 -> Demux/1
  Demux/1 -> Product/2
  Demux/2 -> Product1/2
  Demux/3 -> Product2/2
  [MPCC_f32SwitchingPeriod] -> Product2/1, Product1/1, Product/1
  Product/1 -> MPCC_f32Time1/1
  Product1/1 -> MPCC_f32Time2/1
  Product2/1 -> MPCC_f32Time0/1
  Demux/4 -> MPCC_u8ModulationSector/1

== system Copy_of_AB_Final_of_MPC_Bandwidth_Result/Subsystem1/SOGI 1st/Integrator ==
  In : Inport
  Delay1 : Delay  DelayLength=1
  Delay2 : Delay  DelayLength=1
  Delay3 : Delay  DelayLength=1
  Gain : Gain  Gain=100e-6/12
  Gain1 : Gain  Gain=23
  Gain2 : Gain  Gain=16
  Gain3 : Gain  Gain=5
  Sum : Sum  Inputs=|+-
  Sum1 : Sum  Inputs=|++
  Sum2 : Sum  Inputs=|++
  Out : Outport
  wires:
  Delay2/1 -> Gain2/1, Delay3/1
  Delay1/1 -> Sum2/2, Gain1/1, Delay2/1
  Delay3/1 -> Gain3/1
  Gain2/1 -> Sum/2
  Gain1/1 -> Sum/1
  Gain3/1 -> Sum1/2
  Sum/1 -> Sum1/1
  Gain/1 -> Sum2/1
  Sum2/1 -> Delay1/1
  In/1 -> Gain/1
  Sum1/1 -> Out/1

== system Copy_of_AB_Final_of_MPC_Bandwidth_Result/Subsystem1/SOGI 1st/Integrator1 ==
  In : Inport
  Delay1 : Delay  DelayLength=1
  Delay2 : Delay  DelayLength=1
  Delay3 : Delay  DelayLength=1
  Gain : Gain  Gain=100e-6/12
  Gain1 : Gain  Gain=23
  Gain2 : Gain  Gain=16
  Gain3 : Gain  Gain=5
  Sum : Sum  Inputs=|+-
  Sum1 : Sum  Inputs=|++
  Sum2 : Sum  Inputs=|++
  Out : Outport
  wires:
  Delay2/1 -> Gain2/1, Delay3/1
  Delay1/1 -> Sum2/2, Gain1/1, Delay2/1
  Delay3/1 -> Gain3/1
  Gain2/1 -> Sum/2
  Gain1/1 -> Sum/1
  Gain3/1 -> Sum1/2
  Sum/1 -> Sum1/1
  Gain/1 -> Sum2/1
  Sum2/1 -> Delay1/1
  In/1 -> Gain/1
  Sum1/1 -> Out/1

== system Copy_of_AB_Final_of_MPC_Bandwidth_Result/Subsystem1/SOGI 1st/Integrator2 ==
  In : Inport
  Delay1 : Delay  DelayLength=1
  Delay2 : Delay  DelayLength=1
  Delay3 : Delay  DelayLength=1
  Gain : Gain  Gain=100e-6/12
  Gain1 : Gain  Gain=23
  Gain2 : Gain  Gain=16
  Gain3 : Gain  Gain=5
  Sum : Sum  Inputs=|+-
  Sum1 : Sum  Inputs=|++
  Sum2 : Sum  Inputs=|++
  Out : Outport
  wires:
  In/1 -> Gain/1
  Delay2/1 -> Gain2/1, Delay3/1
  Delay1/1 -> Sum2/2, Gain1/1, Delay2/1
  Delay3/1 -> Gain3/1
  Gain2/1 -> Sum/2
  Gain1/1 -> Sum/1
  Gain3/1 -> Sum1/2
  Sum/1 -> Sum1/1
  Sum1/1 -> Out/1
  Gain/1 -> Sum2/1
  Sum2/1 -> Delay1/1

== system Copy_of_AB_Final_of_MPC_Bandwidth_Result/Subsystem1/Subsystem1/CodeGeneration ==
  Input : Inport
  Add : Sum  Inputs=+-  OutDataTypeStr=Inherit: Same as first input
  Demux2 : Demux  Outputs=2
  Index Vector : MultiPortSwitch  Inputs=1  SaturateOnIntegerOverflow=off  InputSameDT=off
  SCI Transmit : c280xlib/SCI Transmit  sciModule=A  dataHead=''  dataTail=''  blockingMode=on  outputStatus=off
  While Iterator : WhileIterator  MaxIters=-1  WhileBlockType=do-while  ShowIterationPort=on  OutputDataType=int16
  wires:
  While Iterator/1 -> Add/2, Index Vector/1
  Demux2/1 -> Index Vector/2
  Index Vector/1 -> SCI Transmit/1
  Add/1 -> While Iterator/1
  Demux2/2 -> Add/1
  Input/1 -> Demux2/1

== system Copy_of_AB_Final_of_MPC_Bandwidth_Result/Subsystem1/Subsystem1/Data ==
  Data : Inport
  Data_width : Inport  Port=2
  Action Port : ActionPort  ActionPortLabel=else
  Mux : Mux  Inputs=2
  Start : Constant  Value=hex2dec('0000')  OutDataTypeStr=uint16
  Data_out : Outport  VectorParamsAs1DForOutWhenUnconnected=off
  Iteration : Outport  Port=2  VectorParamsAs1DForOutWhenUnconnected=off
  wires:
  Start/1 -> Mux/2
  Mux/1 -> Data_out/1
  Data/1 -> Mux/1
  Data_width/1 -> Iteration/1

== system Copy_of_AB_Final_of_MPC_Bandwidth_Result/Subsystem1/Subsystem1/Data_Conditioning ==
  In1 : Inport
  Data Type Conversion3 : DataTypeConversion  OutDataTypeStr=uint16  ConvertRealWorld=Stored Integer (SI)  SaturateOnIntegerOverflow=off  RndMeth=Floor
  Out1 : Outport  VectorParamsAs1DForOutWhenUnconnected=off
  wires:
  Data Type Conversion3/1 -> Out1/1
  In1/1 -> Data Type Conversion3/1

== system Copy_of_AB_Final_of_MPC_Bandwidth_Result/Subsystem1/Subsystem1/End ==
  Data : Inport
  Data_width : Inport  Port=2
  Action Port : ActionPort  ActionPortLabel=elseif(u1 == 599)
  Bias : Bias  Bias=1  SaturateOnIntegerOverflow=off
  Mux : Mux  Inputs=2
  Start : Constant  Value=hex2dec('4545')  OutDataTypeStr=uint16
  Data_out : Outport  VectorParamsAs1DForOutWhenUnconnected=off
  Iteration : Outport  Port=2  VectorParamsAs1DForOutWhenUnconnected=off
  wires:
  Mux/1 -> Data_out/1
  Data_width/1 -> Bias/1
  Start/1 -> Mux/2
  Bias/1 -> Iteration/1
  Data/1 -> Mux/1

== system Copy_of_AB_Final_of_MPC_Bandwidth_Result/Subsystem1/Subsystem1/Start ==
  Data : Inport
  Data_width : Inport  Port=2
  Action Port : ActionPort  ActionPortLabel=if(u1 == 0)
  Bias : Bias  Bias=1  SaturateOnIntegerOverflow=off
  End : Constant  Value=hex2dec('5353')  OutDataTypeStr=uint16
  Mux : Mux  Inputs=2
  Data_out : Outport  VectorParamsAs1DForOutWhenUnconnected=off
  Iteration : Outport  Port=2  VectorParamsAs1DForOutWhenUnconnected=off
  wires:
  End/1 -> Mux/1
  Mux/1 -> Data_out/1
  Data_width/1 -> Bias/1
  Bias/1 -> Iteration/1
  Data/1 -> Mux/2

== system Copy_of_AB_Final_of_MPC_Bandwidth_Result/Subsystem1/Subsystem2/CodeGeneration ==
  Input : Inport
  Add : Sum  Inputs=+-  OutDataTypeStr=Inherit: Same as first input
  Demux2 : Demux  Outputs=2
  Index Vector : MultiPortSwitch  Inputs=1  SaturateOnIntegerOverflow=off  InputSameDT=off
  SCI Transmit : c280xlib/SCI Transmit  sciModule=A  dataHead=''  dataTail=''  blockingMode=on  outputStatus=off
  While Iterator : WhileIterator  MaxIters=-1  WhileBlockType=do-while  ShowIterationPort=on  OutputDataType=int16
  wires:
  While Iterator/1 -> Add/2, Index Vector/1
  Demux2/1 -> Index Vector/2
  Index Vector/1 -> SCI Transmit/1
  Add/1 -> While Iterator/1
  Demux2/2 -> Add/1
  Input/1 -> Demux2/1

== system Copy_of_AB_Final_of_MPC_Bandwidth_Result/Subsystem1/Subsystem2/Data ==
  Data : Inport
  Data_width : Inport  Port=2
  Action Port : ActionPort  ActionPortLabel=else
  Mux : Mux  Inputs=2
  Start : Constant  Value=hex2dec('0000')  OutDataTypeStr=uint16
  Data_out : Outport  VectorParamsAs1DForOutWhenUnconnected=off
  Iteration : Outport  Port=2  VectorParamsAs1DForOutWhenUnconnected=off
  wires:
  Start/1 -> Mux/2
  Mux/1 -> Data_out/1
  Data/1 -> Mux/1
  Data_width/1 -> Iteration/1

== system Copy_of_AB_Final_of_MPC_Bandwidth_Result/Subsystem1/Subsystem2/Data_Conditioning ==
  In1 : Inport
  Data Type Conversion3 : DataTypeConversion  OutDataTypeStr=uint16  ConvertRealWorld=Stored Integer (SI)  SaturateOnIntegerOverflow=off  RndMeth=Floor
  Out1 : Outport  VectorParamsAs1DForOutWhenUnconnected=off
  wires:
  Data Type Conversion3/1 -> Out1/1
  In1/1 -> Data Type Conversion3/1

== system Copy_of_AB_Final_of_MPC_Bandwidth_Result/Subsystem1/Subsystem2/End ==
  Data : Inport
  Data_width : Inport  Port=2
  Action Port : ActionPort  ActionPortLabel=elseif(u1 == 599)
  Bias : Bias  Bias=1  SaturateOnIntegerOverflow=off
  Mux : Mux  Inputs=2
  Start : Constant  Value=hex2dec('4545')  OutDataTypeStr=uint16
  Data_out : Outport  VectorParamsAs1DForOutWhenUnconnected=off
  Iteration : Outport  Port=2  VectorParamsAs1DForOutWhenUnconnected=off
  wires:
  Mux/1 -> Data_out/1
  Data_width/1 -> Bias/1
  Start/1 -> Mux/2
  Bias/1 -> Iteration/1
  Data/1 -> Mux/1

== system Copy_of_AB_Final_of_MPC_Bandwidth_Result/Subsystem1/Subsystem2/Start ==
  Data : Inport
  Data_width : Inport  Port=2
  Action Port : ActionPort  ActionPortLabel=if(u1 == 0)
  Bias : Bias  Bias=1  SaturateOnIntegerOverflow=off
  End : Constant  Value=hex2dec('5353')  OutDataTypeStr=uint16
  Mux : Mux  Inputs=2
  Data_out : Outport  VectorParamsAs1DForOutWhenUnconnected=off
  Iteration : Outport  Port=2  VectorParamsAs1DForOutWhenUnconnected=off
  wires:
  End/1 -> Mux/1
  Mux/1 -> Data_out/1
  Data_width/1 -> Bias/1
  Bias/1 -> Iteration/1
  Data/1 -> Mux/2

== system Copy_of_AB_Final_of_MPC_Bandwidth_Result/Subsystem1/VoltageReferenceCalculation/ElectricalAngleCompensation ==
  MPCC_f32SamplingPeriod : Inport
  MPCC_f32AngularFrequency : Inport  Port=2
  MPCC_f32ElectricalAngle : Inport  Port=3
  Add1 : Sum
  Gain1 : Gain  Gain=1.5
  Product1 : Product
  MPCC_f32ElectricalAngle_K_1 : Outport
  wires:
  MPCC_f32AngularFrequency/1 -> Product1/2
  Product1/1 -> Gain1/1
  MPCC_f32SamplingPeriod/1 -> Product1/1
  Gain1/1 -> Add1/1
  MPCC_f32ElectricalAngle/1 -> Add1/2
  Add1/1 -> MPCC_f32ElectricalAngle_K_1/1

== system Copy_of_AB_Final_of_MPC_Bandwidth_Result/Subsystem1/VoltageReferenceCalculation/PredictiveTermsCalculation ==
  MPCC_f32RGrid : Inport
  MPCC_f32LGrid : Inport  Port=2
  MPCC_f32SamplingPeriod : Inport  Port=3
  MPCC_f32AngularFrequency : Inport  Port=4
  Add : Sum
  Constant : Constant  Value=single(1)
  Divide : Product  Inputs=*/  RndMeth=Zero  SaturateOnIntegerOverflow=on
  Divide1 : Product  Inputs=*/  RndMeth=Zero  SaturateOnIntegerOverflow=on
  Gain : Gain  Gain=-1
  Product : Product
  Product1 : Product
  MPCC_f32Predictionterm_A : Outport
  MPCC_f32Predictionterm_B : Outport  Port=2
  MPCC_f32Predictionterm_C : Outport  Port=3
  wires:
  Divide/1 -> Add/1
  Gain/1 -> Product/1
  MPCC_f32AngularFrequency/1 -> Product1/2
  [MPCC_f32LGrid] -> Divide1/2
  MPCC_f32SamplingPeriod/1 -> Product/2, [MPCC_f32SamplingPeriod]
  Divide1/1 -> MPCC_f32Predictionterm_B/1
  [MPCC_f32SamplingPeriod] -> Divide1/1
  Product1/1 -> MPCC_f32Predictionterm_C/1
  Constant/1 -> Add/2
  MPCC_f32RGrid/1 -> Gain/1
  MPCC_f32LGrid/1 -> [MPCC_f32LGrid], Divide/2
  [MPCC_f32SamplingPeriod] -> Product1/1
  Product/1 -> Divide/1
  Add/1 -> MPCC_f32Predictionterm_A/1

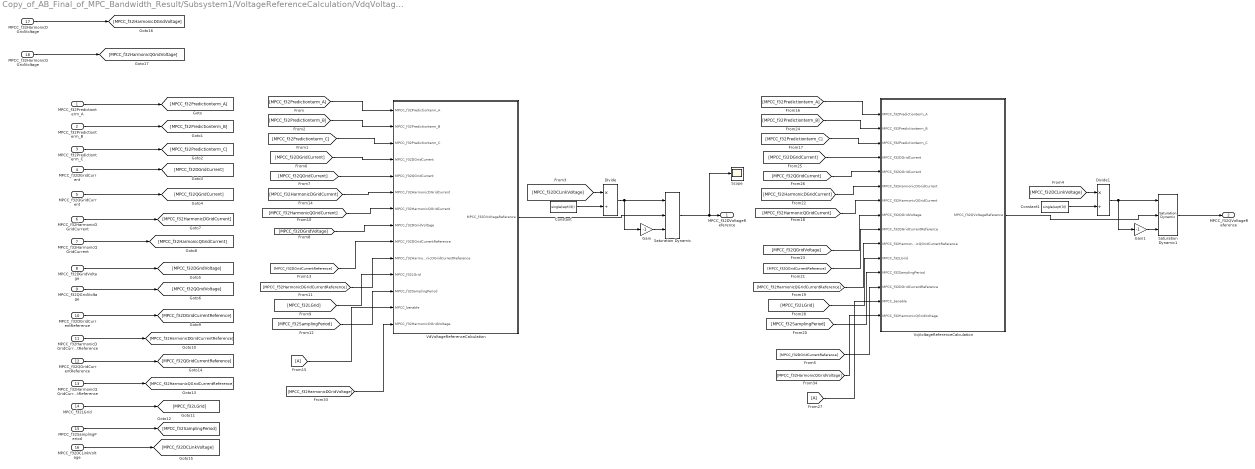
== system Copy_of_AB_Final_of_MPC_Bandwidth_Result/Subsystem1/VoltageReferenceCalculation/VdqVoltageReferenceCalculation ==
  MPCC_f32Predictionterm_A : Inport
  MPCC_f32Predictionterm_B : Inport  Port=2
  MPCC_f32Predictionterm_C : Inport  Port=3
  MPCC_f32DGridCurrent : Inport  Port=4
  MPCC_f32QGridCurrent : Inport  Port=5
  MPCC_f32HarmonicDGridCurrent : Inport  Port=6
  MPCC_f32HarmonicQGridCurrent : Inport  Port=7
  MPCC_f32DGridVoltage : Inport  Port=8
  MPCC_f32QGridVoltage : Inport  Port=9
  MPCC_f32DGridCurrentReference : Inport  Port=10
  MPCC_f32HarmonicDGridCurrentReference : Inport  Port=11
  MPCC_f32QGridCurrentReference : Inport  Port=12
  MPCC_f32HarmonicQGridCurrentReference : Inport  Port=13
  MPCC_f32LGrid : Inport  Port=14
  MPCC_f32SamplingPeriod : Inport  Port=15
  MPCC_f32DCLinkVoltage : Inport  Port=16
  MPCC_f32HarmonicDGridVoltage : Inport  Port=17
  MPCC_f32HarmonicQGridVoltage : Inport  Port=18
  Constant : Constant  Value=single(sqrt(3))
  Constant1 : Constant  Value=single(sqrt(3))
  Divide : Product  Inputs=*/  RndMeth=Zero  SaturateOnIntegerOverflow=on
  Divide1 : Product  Inputs=*/  RndMeth=Zero  SaturateOnIntegerOverflow=on
  From15 : From
  From27 : From
  Gain : Gain  Gain=-1
  Gain1 : Gain  Gain=-1
  Saturation Dynamic : simulink/Discontinuities/Saturation Dynamic  OutMin=[]  OutMax=[]  OutDataTypeStr=Inherit: Same as second input  OutDataType=fixdt(1, 16)  OutScaling=2^-10  DoSatur=off
  Saturation Dynamic1 : simulink/Discontinuities/Saturation Dynamic  OutMin=[]  OutMax=[]  OutDataTypeStr=Inherit: Same as second input  OutDataType=fixdt(1, 16)  OutScaling=2^-10  DoSatur=off
  Scope : Scope
  VdVoltageReferenceCalculation : Subsystem
  VqVoltageReferenceCalculation : Subsystem
  MPCC_f32DVoltageReference : Outport
  MPCC_f32QVoltageReference : Outport  Port=2
  wires:
  [MPCC_f32Predictionterm_A] -> VdVoltageReferenceCalculation/1(MPCC_f32Predictionterm_A)
  [MPCC_f32Predictionterm_B] -> VdVoltageReferenceCalculation/2(MPCC_f32Predictionterm_B)
  [MPCC_f32Predictionterm_C] -> VdVoltageReferenceCalculation/3(MPCC_f32Predictionterm_C)
  MPCC_f32LGrid/1 -> [MPCC_f32LGrid]
  MPCC_f32DGridVoltage/1 -> [MPCC_f32DGridVoltage]
  MPCC_f32Predictionterm_A/1 -> [MPCC_f32Predictionterm_A]
  MPCC_f32QGridVoltage/1 -> [MPCC_f32QGridVoltage]
  MPCC_f32DGridCurrentReference/1 -> [MPCC_f32DGridCurrentReference]
  MPCC_f32Predictionterm_C/1 -> [MPCC_f32Predictionterm_C]
  MPCC_f32HarmonicQGridCurrent/1 -> [MPCC_f32HarmonicQGridCurrent]
  MPCC_f32Predictionterm_B/1 -> [MPCC_f32Predictionterm_B]
  MPCC_f32DGridCurrent/1 -> [MPCC_f32DGridCurrent]
  MPCC_f32HarmonicDGridCurrent/1 -> [MPCC_f32HarmonicDGridCurrent]
  MPCC_f32HarmonicDGridCurrentReference/1 -> [MPCC_f32HarmonicDGridCurrentReference]
  MPCC_f32QGridCurrent/1 -> [MPCC_f32QGridCurrent]
  MPCC_f32SamplingPeriod/1 -> [MPCC_f32SamplingPeriod]
  [MPCC_f32DGridCurrent] -> VdVoltageReferenceCalculation/4(MPCC_f32DGridCurrent)
  [MPCC_f32QGridCurrent] -> VdVoltageReferenceCalculation/5(MPCC_f32QGridCurrent)
  [MPCC_f32HarmonicDGridCurrent] -> VdVoltageReferenceCalculation/6(MPCC_f32HarmonicDGridCurrent)
  [MPCC_f32HarmonicQGridCurrent] -> VdVoltageReferenceCalculation/7(MPCC_f32HarmonicQGridCurrent)
  [MPCC_f32DGridVoltage] -> VdVoltageReferenceCalculation/8(MPCC_f32DGridVoltage)
  [MPCC_f32DGridCurrentReference] -> VdVoltageReferenceCalculation/9(MPCC_f32DGridCurrentReference)
  [MPCC_f32HarmonicDGridCurrentReference] -> VdVoltageReferenceCalculation/10(MPCC_f32HarmonicDGridCurrentReference)
  [MPCC_f32LGrid] -> VdVoltageReferenceCalculation/11(MPCC_f32LGrid)
  [MPCC_f32SamplingPeriod] -> VdVoltageReferenceCalculation/12(MPCC_f32SamplingPeriod)
  [MPCC_f32Predictionterm_B] -> VqVoltageReferenceCalculation/2(MPCC_f32Predictionterm_B)
  [MPCC_f32LGrid] -> VqVoltageReferenceCalculation/11(MPCC_f32LGrid)
  [MPCC_f32SamplingPeriod] -> VqVoltageReferenceCalculation/12(MPCC_f32SamplingPeriod)
  [MPCC_f32QGridVoltage] -> VqVoltageReferenceCalculation/8(MPCC_f32QGridVoltage)
  [MPCC_f32Predictionterm_A] -> VqVoltageReferenceCalculation/1(MPCC_f32Predictionterm_A)
  [MPCC_f32HarmonicDGridCurrent] -> VqVoltageReferenceCalculation/6(MPCC_f32HarmonicDGridCurrent)
  [MPCC_f32HarmonicQGridCurrentReference] -> VqVoltageReferenceCalculation/10(MPCC_f32HarmonicQGridCurrentReference)
  [MPCC_f32QGridCurrent] -> VqVoltageReferenceCalculation/5(MPCC_f32QGridCurrent)
  [MPCC_f32Predictionterm_C] -> VqVoltageReferenceCalculation/3(MPCC_f32Predictionterm_C)
  [MPCC_f32QGridCurrentReference] -> VqVoltageReferenceCalculation/9(MPCC_f32QGridCurrentReference)
  [MPCC_f32DGridCurrent] -> VqVoltageReferenceCalculation/4(MPCC_f32DGridCurrent)
  [MPCC_f32HarmonicQGridCurrent] -> VqVoltageReferenceCalculation/7(MPCC_f32HarmonicQGridCurrent)
  MPCC_f32QGridCurrentReference/1 -> [MPCC_f32QGridCurrentReference]
  MPCC_f32HarmonicQGridCurrentReference/1 -> [MPCC_f32HarmonicQGridCurrentReference]
  MPCC_f32DCLinkVoltage/1 -> [MPCC_f32DCLinkVoltage]
  [MPCC_f32DCLinkVoltage] -> Divide/1
  Constant/1 -> Divide/2
  Divide/1 -> Gain/1, Saturation Dynamic/1
  Gain/1 -> Saturation Dynamic/3
  Saturation Dynamic/1 -> Scope/1, MPCC_f32DVoltageReference/1
  [MPCC_f32DCLinkVoltage] -> Divide1/1
  Constant1/1 -> Divide1/2
  Gain1/1 -> Saturation Dynamic1/3
  Divide1/1 -> Gain1/1, Saturation Dynamic1/1
  Saturation Dynamic1/1 -> MPCC_f32QVoltageReference/1
  [MPCC_f32DGridCurrentReference] -> VqVoltageReferenceCalculation/13(MPCC_f32DGridCurrentReference)
  From15/1 -> VdVoltageReferenceCalculation/13(MPCC_benable)
  From27/1 -> VqVoltageReferenceCalculation/14(MPCC_benable)
  MPCC_f32HarmonicDGridVoltage/1 -> [MPCC_f32HarmonicDGridVoltage]
  MPCC_f32HarmonicQGridVoltage/1 -> [MPCC_f32HarmonicQGridVoltage]
  VdVoltageReferenceCalculation/1(MPCC_f32DVoltageReference) -> Saturation Dynamic/2
  VqVoltageReferenceCalculation/1(MPCC_f32QVoltageReference) -> Saturation Dynamic1/2
  [MPCC_f32HarmonicDGridVoltage] -> VdVoltageReferenceCalculation/14(MPCC_f32HarmonicDGridVoltage)
  [MPCC_f32HarmonicQGridVoltage] -> VqVoltageReferenceCalculation/15(MPCC_f32HarmonicQGridVoltage)

== system Copy_of_AB_Final_of_MPC_Bandwidth_Result/Subsystem1/dq_abc1/Subsystem6 ==
  In1 : Inport
  In2 : Inport  Port=2
  theta : Inport  Port=3
  Add{,1,3..4} (4 alike) : Sum  Inputs=+-
  Add2 : Sum
  Constant : Constant  Value=2*pi/3
  Cos : Trigonometry  Operator=cos
  Cos1 : Trigonometry
  Cos2 : Trigonometry  Operator=cos
  Cos3 : Trigonometry
  Cos4 : Trigonometry
  Cos5 : Trigonometry  Operator=cos
  Product{,1..5} (6 alike) : Product
  Ia : Outport
  Ib : Outport  Port=2
  Ic : Outport  Port=3
  wires:
  theta/1 -> Add2/2, Add3/1, Cos1/1, Cos/1
  In1/1 -> [d]
  In2/1 -> [q]
  [d] -> Product/1
  Cos/1 -> [cosine]
  Cos1/1 -> [sinee]
  [cosine] -> Product/2
  [q] -> Product1/1
  [sinee] -> Product1/2
  Product/1 -> Add/1
  Product1/1 -> Add/2
  Add/1 -> Ia/1
  Constant/1 -> Add3/2, Add2/1
  Add2/1 -> Cos4/1, Cos2/1
  Add3/1 -> Cos5/1, Cos3/1
  Add1/1 -> Ib/1
  [d] -> Product2/1
  Cos3/1 -> Product3/2
  Product3/1 -> Add1/2
  [q] -> Product3/1
  Product2/1 -> Add1/1
  Cos5/1 -> Product2/2
  [q] -> Product5/1
  [d] -> Product4/1
  Product4/1 -> Add4/1
  Add4/1 -> Ic/1
  Cos4/1 -> Product5/2
  Product5/1 -> Add4/2
  Cos2/1 -> Product4/2

== system Copy_of_AB_Final_of_MPC_Bandwidth_Result/Subsystem3/PLL2/Clarke Transformation1 ==
  va : Inport
  vb : Inport  Port=2
  vc : Inport  Port=3
  Gain1 : Gain  Gain=0.5
  Gain2 : Gain  Gain=0.5
  Gain3 : Gain  Gain=2/3
  Gain4 : Gain  Gain=2/3
  Gain5 : Gain  Gain=sqrt(3)/2
  Sum : Sum  Inputs=+--
  Sum1 : Sum  Inputs=+-
  I_alpha : Outport
  I_beta : Outport  Port=2
  wires:
  Gain1/1 -> Sum/3
  Gain2/1 -> Sum/2
  Gain4/1 -> I_beta/1
  Sum/1 -> Gain3/1
  Gain3/1 -> I_alpha/1
  va/1 -> Sum/1
  Sum1/1 -> Gain5/1
  vc/1 -> Gain1/1, Sum1/2
  Gain5/1 -> Gain4/1
  vb/1 -> Gain2/1, Sum1/1
